simulink model "bh_3LINK_NEWTON_model_write_hello"  (R2022b)
settings: Solver=ode15s  StartTime=0.0  StopTime=30  FixedStep=0.001  RelTol=1e-6  EnableMultiTasking=on
libraries: sm_lib x1
settings Model: Creator=bhorton  LastModifiedBy=bhorton
settings SolverCC: ZeroCrossAlgorithm=Adaptive  AlgebraicLoopSolver=TrustRegion
settings DataIOCC: ReturnWorkspaceOutputs=off
settings OptimizationCC: BlockReduction=off  LifeSpan=inf
settings DebuggingCC: UnconnectedInputMsg=warning  UnconnectedOutputMsg=warning  UnconnectedLineMsg=warning  SFUnexpectedBacktrackingDiag=warning  SFNoUnconditionalDefaultTransitionDiag=warning  SFExecutionAtInitializationDiag=none  SFMachineParentedDataDiag=warning  ArithmeticOperatorsInVariantConditions=warning
settings ModelReferenceCC: EnableRefExpFcnMdlSchedulingChecks=on
settings SFSimCC: SimUseLocalCustomCode=off  CustomCodeUndefinedFunction=UseInterfaceOnly
settings RTWCC: RTWUseLocalCustomCode=off  DLArmComputeVersion=19.05
settings CodeAppCC: StateflowObjectComments=on
settings GRTTargetCC: TargetLangStandard=C89/C90 (ANSI)
settings ConfigComp: CovMetricSettings=dw  CovSaveCumulativeToWorkspaceVar=on  CovSaveSingleToWorkspaceVar=on  CovExternalEMLEnable=off
settings SimscapeCC: SimscapeNormalizeSystem=off  SimscapeLogType=all  SimscapeLogDataHistory=10000
settings ExplorerConfigSet: InternalSimMechanicsExplorerSettings="<ExplorerConfiguration><canonicalview>default</canonicalview><AnimationSetting><BasePlaybackSpeed>1.0</BasePlaybackSpeed><PlaybackSpeedFactor>1.0</PlaybackSpeedFactor></AnimationSetting><TilePanel><TileInfo><Tiles Columns=\"1\" Count=\"1\" Rows=\"1\"><Column Weight=\"1\"/><Row Weight=\"1\"/><Tile Height=\"1\" Width=\"1\" X=\"0\" Y=\"0\"/></Tiles></TileInfo><SceneInfo><SceneViewer><BGColor><R>0.60000002384185791</R><G>0.60000002384185791</G><B>0.60000002384185791</B></BGColor><Camera><DoPerspective>off</DoPerspective><Position><X>0.59337591503002618</X><Y>0.770028921233025243</Y><Z>1.16558506746291179</Z></Position><Center><X>0.554818716269093848</X><Y>0.595850240273192444</Y><Z>-0.00768042407463245119</Z></Center><Up><X>0.010293767731727228</X><Y>0.989057625734068191</Y><Z>-0.147170144129760788</Z></Up><ViewLimDist>1</ViewLimDist><YLim>0.684058578463238476</YLim><XLim>1.00632617542814184</XLim></Camera></SceneViewer></SceneInfo></TilePanel><MechEditorPanel><Cameras/><GfxPanelCameraMap/><VideoCreator><PlaybackSpeedRatio>1.0</PlaybackSpeedRatio><FrameRate>24</FrameRate><VideoFormat>MPEG-4</VideoFormat><FrameSize>[400 400]</FrameSize></VideoCreator></MechEditorPanel></ExplorerConfiguration>"

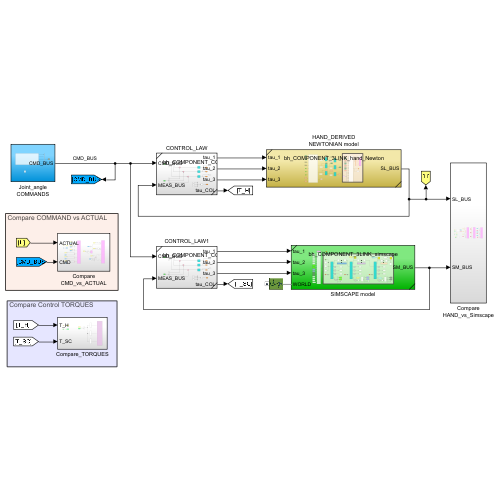
[thumbnail: Simulink's stored preview of the top-level diagram]
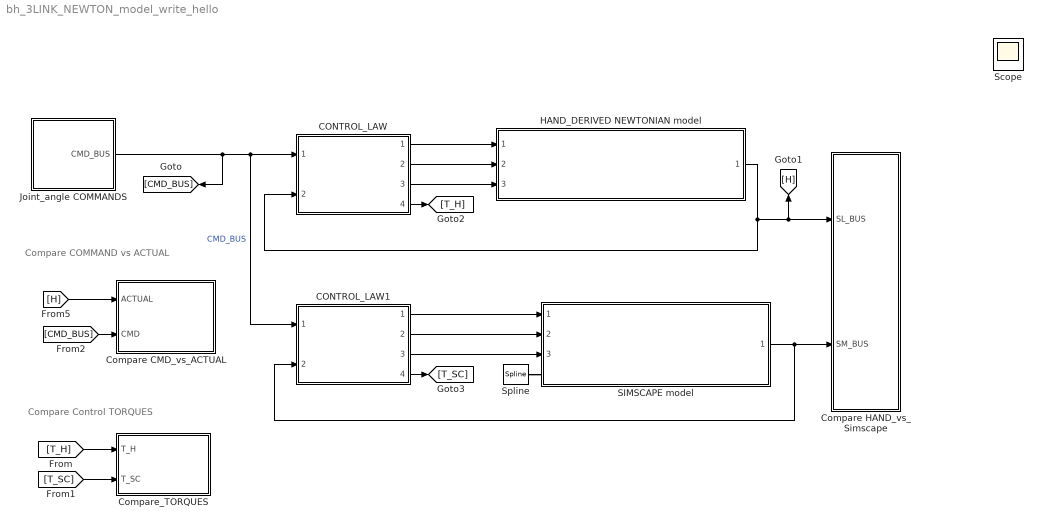
== system bh_3LINK_NEWTON_model_write_hello ==
  note: Compare Control TORQUES
  note: Compare COMMAND vs ACTUAL
  CONTROL_LAW : Subsystem  ReferencedSubsystem=bh_COMPONENT_CONTROL_LAW
  CONTROL_LAW1 : Subsystem  ReferencedSubsystem=bh_COMPONENT_CONTROL_LAW
  Compare CMD_vs_ACTUAL : Subsystem
  Compare HAND_vs_Simscape : Subsystem
  Compare_TORQUES : Subsystem
  HAND_DERIVED NEWTONIAN model : Subsystem  ReferencedSubsystem=bh_COMPONENT_3LINK_hand_Newton
  Joint_angle COMMANDS : Subsystem
  SIMSCAPE model : Subsystem  ReferencedSubsystem=bh_COMPONENT_3LINK_simscape
  Spline : sm_lib/Curves and Surfaces/Spline  GraphicAmbientColor=[0.15 0.15 0.15 1.0]  GraphicDiffuseColor=[0.0 1.0 0.0]  DataPoints=the_EE.XYZ_spline  DataPointsUnits=m  GraphicEmissiveColor=[0.0 0.0 0.0 1.0]  EndConditionType=Natural  MarkerShape=Sphere  MarkerSize=10  GraphicType=FromGeometry  GraphicOpacity=1.0  GraphicShininess=75  GraphicSpecularColor=[0.5 0.5 0.5 1.0]  GraphicVisPropType=SimpleVisualProperties
  Scope : Scope
  wires:
  SIMSCAPE model/1 -> CONTROL_LAW1/2, Compare HAND_vs_Simscape/2(SM_BUS)
  HAND_DERIVED NEWTONIAN model/1 -> Compare HAND_vs_Simscape/1(SL_BUS), [H], CONTROL_LAW/2
  Joint_angle COMMANDS/1(CMD_BUS) -> [CMD_BUS], CONTROL_LAW1/1, CONTROL_LAW/1  "CMD_BUS"
  CONTROL_LAW/1 -> HAND_DERIVED NEWTONIAN model/1
  CONTROL_LAW/2 -> HAND_DERIVED NEWTONIAN model/2
  CONTROL_LAW/3 -> HAND_DERIVED NEWTONIAN model/3
  CONTROL_LAW1/1 -> SIMSCAPE model/1
  CONTROL_LAW1/2 -> SIMSCAPE model/2
  CONTROL_LAW1/3 -> SIMSCAPE model/3
  [CMD_BUS] -> Compare CMD_vs_ACTUAL/2(CMD)
  [H] -> Compare CMD_vs_ACTUAL/1(ACTUAL)
  CONTROL_LAW/4 -> [T_H]
  CONTROL_LAW1/4 -> [T_SC]
  [T_SC] -> Compare_TORQUES/2(T_SC)
  [T_H] -> Compare_TORQUES/1(T_H)
  connections:
  Spline/LConn1 -- SIMSCAPE model/LConn1

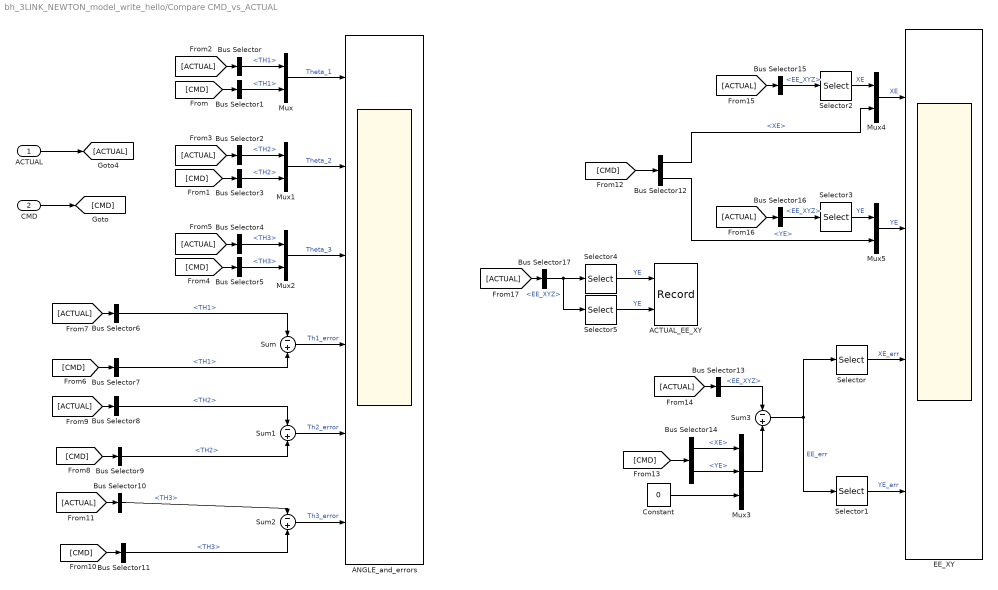
== system bh_3LINK_NEWTON_model_write_hello/Compare CMD_vs_ACTUAL ==
  ACTUAL : Inport
  CMD : Inport  Port=2
  ACTUAL_EE_XY : Record  FileSettingsInternal="{\"entries\":[{\"content\":{\"excelSettings\":{\"content\":{},\"type\":\"Streamout.ExcelSettings\"}},\"type\":\"Streamout.FileSettingStorage\",\"uuid\":\"47bc9f06-3dd7-4c30-9e65-8a4f675568b5\"}],\"packageUris\":[\"http://schema.mathworks.com/mf0/streamout_blocks/R2020a\"],\"version\":\"1.0\"}"  Layout=[1 1]  SignalsInternal="{\"entries\":[{\"content\":{\"signals\":[{\"content\":{\"blockPath\":[\"bh_3LINK_NEWTON_model_write_hello/Compare CMD_vs_ACTUAL/ACTUAL_EE_XY\"],\"channel\":[],\"dimensions\":[1],\"domain\":\"bh_3LINK_NEWTON_model_write_hello/Compare CMD_vs_ACTUAL/ACTUAL_EE_XY\",\"lineColor\":\"#ff6929\",\"plots\":[],\"port\":1,\"sid\":[],\"signalID\":3905,\"signalName\":\"YE\"},\"type\":\"RecordBlkView.Signal\",\"uuid\":\"7d422940-e755-4ad5-abac-504df8c7a942\"},{\"content\":{\"blockPath\":[\"bh_3LINK_NEWTON_model_write_hello/Compare CMD_vs_ACTUAL/ACTUAL_EE_XY\"],\"channel\":[],\"dimensions\":[1],\"domain\":\"bh_3LINK_NEWTON_model_write_hello/Compare CMD_vs_ACTUAL/ACTUAL_EE_XY\",\"lineColor\":\"#b746ff\",\"plots\":[],\"port\":2,\"sid\":[],\"signalID\":3908,\"signalName\":\"YE\"},\"type\":\"RecordBlkView.Signal\",\"uuid\":\"e4267c01-9c27-4ae9-8327-b877059776d0\"}]},\"type\":\"RecordBlkView.InputSignals\",\"uuid\":\"38542130-8fed-4a5c-a1bf-593c8935b6a0\"}],\"packageUris\":[\"http://schema.mathworks.com/mf0/streamout_blocks/R2020a\"],\"version\":\"1.0\"}"  VisualizationBindings="{\"xyplotplugin\":{\"info\":[{\"series\":[],\"subplotID\":1}]}}"  CompatibilityTag=XY  st=-1
  ANGLE_and_errors : Scope  NumInputPorts=6
  Bus Selector{,1,6..7} (4 alike) : BusSelector  OutputSignals=TH1
  Bus Selector{4..5,10..11} (4 alike) : BusSelector  OutputSignals=TH3
  Bus Selector12 : BusSelector  OutputSignals=XE,YE
  Bus Selector{13,15..17} (4 alike) : BusSelector  OutputSignals=EE_XYZ
  Bus Selector14 : BusSelector  OutputSignals=XE,YE
  Bus Selector{2..3,8..9} (4 alike) : BusSelector  OutputSignals=TH2
  Constant : Constant  Value=0
  EE_XY : Scope  NumInputPorts=4
  Mux{,1..2,4..5} (5 alike) : Mux  Inputs=2
  Mux3 : Mux  Inputs=3
  Selector : Selector  InputPortWidth=3  IndexOptions=Index vector (dialog)  Indices=1  OutputSizes=1
  Selector1 : Selector  InputPortWidth=3  IndexOptions=Index vector (dialog)  Indices=2  OutputSizes=1
  Selector2 : Selector  InputPortWidth=3  IndexOptions=Index vector (dialog)  Indices=1  OutputSizes=1
  Selector3 : Selector  InputPortWidth=3  IndexOptions=Index vector (dialog)  Indices=2  OutputSizes=1
  Selector4 : Selector  InputPortWidth=3  IndexOptions=Index vector (dialog)  Indices=1  OutputSizes=1
  Selector5 : Selector  InputPortWidth=3  IndexOptions=Index vector (dialog)  Indices=2  OutputSizes=1
  Sum{,1..3} (4 alike) : Sum  Inputs=-|+
  wires:
  ACTUAL/1 -> [ACTUAL]
  CMD/1 -> [CMD]
  [ACTUAL] -> Bus Selector/1
  Mux/1 -> ANGLE_and_errors/1  "Theta_1"
  Bus Selector/1 -> Mux/1  "<TH1>"
  [CMD] -> Bus Selector1/1
  Bus Selector1/1 -> Mux/2  "<TH1>"
  Bus Selector3/1 -> Mux1/2  "<TH2>"
  [CMD] -> Bus Selector3/1
  Mux1/1 -> ANGLE_and_errors/2  "Theta_2"
  [ACTUAL] -> Bus Selector2/1
  Bus Selector2/1 -> Mux1/1  "<TH2>"
  Mux2/1 -> ANGLE_and_errors/3  "Theta_3"
  [ACTUAL] -> Bus Selector4/1
  [CMD] -> Bus Selector5/1
  Bus Selector5/1 -> Mux2/2  "<TH3>"
  Bus Selector4/1 -> Mux2/1  "<TH3>"
  Sum/1 -> ANGLE_and_errors/4  "Th1_error"
  Sum1/1 -> ANGLE_and_errors/5  "Th2_error"
  Sum2/1 -> ANGLE_and_errors/6  "Th3_error"
  Bus Selector7/1 -> Sum/2  "<TH1>"
  [CMD] -> Bus Selector7/1
  [ACTUAL] -> Bus Selector6/1
  Bus Selector6/1 -> Sum/1  "<TH1>"
  [ACTUAL] -> Bus Selector8/1
  [CMD] -> Bus Selector9/1
  Bus Selector9/1 -> Sum1/2  "<TH2>"
  Bus Selector8/1 -> Sum1/1  "<TH2>"
  Bus Selector11/1 -> Sum2/2  "<TH3>"
  [ACTUAL] -> Bus Selector10/1
  Bus Selector10/1 -> Sum2/1  "<TH3>"
  [CMD] -> Bus Selector11/1
  [CMD] -> Bus Selector12/1
  [ACTUAL] -> Bus Selector13/1
  [CMD] -> Bus Selector14/1
  Sum3/1 -> Selector1/1, Selector/1  "EE_err"
  Selector1/1 -> EE_XY/4  "YE_err"
  Selector/1 -> EE_XY/3  "XE_err"
  Constant/1 -> Mux3/3
  Bus Selector14/1 -> Mux3/1  "<XE>"
  Bus Selector14/2 -> Mux3/2  "<YE>"
  Mux3/1 -> Sum3/2
  Bus Selector13/1 -> Sum3/1  "<EE_XYZ>"
  [ACTUAL] -> Bus Selector15/1
  Bus Selector15/1 -> Selector2/1  "<EE_XYZ>"
  Mux4/1 -> EE_XY/1  "XE"
  Selector2/1 -> Mux4/1  "XE"
  Bus Selector12/1 -> Mux4/2  "<XE>"
  [ACTUAL] -> Bus Selector16/1
  Bus Selector16/1 -> Selector3/1  "<EE_XYZ>"
  Selector3/1 -> Mux5/1  "YE"
  Mux5/1 -> EE_XY/2  "YE"
  Bus Selector12/2 -> Mux5/2  "<YE>"
  [ACTUAL] -> Bus Selector17/1
  Bus Selector17/1 -> Selector5/1, Selector4/1  "<EE_XYZ>"
  Selector5/1 -> ACTUAL_EE_XY/2  "YE"
  Selector4/1 -> ACTUAL_EE_XY/1  "YE"

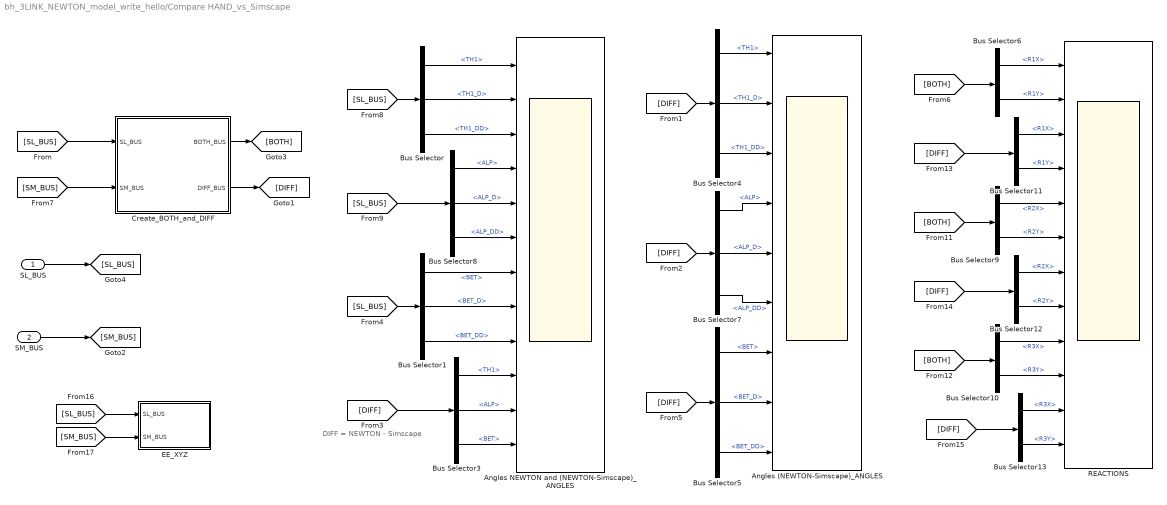
== system bh_3LINK_NEWTON_model_write_hello/Compare HAND_vs_Simscape ==
  note: DIFF = NEWTON - Simscape
  SL_BUS : Inport
  SM_BUS : Inport  Port=2
  Angles (NEWTON-Simscape)_ANGLES : Scope  NumInputPorts=9
  Angles NEWTON and (NEWTON-Simscape)_ANGLES : Scope  NumInputPorts=12
  Bus Selector : BusSelector  OutputSignals=TH1,TH1_D,TH1_DD
  Bus Selector1 : BusSelector  OutputSignals=BET,BET_D,BET_DD
  Bus Selector10 : BusSelector  OutputSignals=R3X,R3Y
  Bus Selector11 : BusSelector  OutputSignals=R1X,R1Y
  Bus Selector12 : BusSelector  OutputSignals=R2X,R2Y
  Bus Selector13 : BusSelector  OutputSignals=R3X,R3Y
  Bus Selector3 : BusSelector  OutputSignals=TH1,ALP,BET
  Bus Selector4 : BusSelector  OutputSignals=TH1,TH1_D,TH1_DD
  Bus Selector5 : BusSelector  OutputSignals=BET,BET_D,BET_DD
  Bus Selector6 : BusSelector  OutputSignals=R1X,R1Y
  Bus Selector7 : BusSelector  OutputSignals=ALP,ALP_D,ALP_DD
  Bus Selector8 : BusSelector  OutputSignals=ALP,ALP_D,ALP_DD
  Bus Selector9 : BusSelector  OutputSignals=R2X,R2Y
  Create_BOTH_and_DIFF : Subsystem
  EE_XYZ : Subsystem
  REACTIONS : Scope  NumInputPorts=12
  wires:
  [SM_BUS] -> Create_BOTH_and_DIFF/2(SM_BUS)
  Bus Selector/3 -> Angles NEWTON and (NEWTON-Simscape)_ANGLES/3  "<TH1_DD>"
  Bus Selector/2 -> Angles NEWTON and (NEWTON-Simscape)_ANGLES/2  "<TH1_D>"
  Bus Selector/1 -> Angles NEWTON and (NEWTON-Simscape)_ANGLES/1  "<TH1>"
  [SL_BUS] -> Create_BOTH_and_DIFF/1(SL_BUS)
  Bus Selector8/1 -> Angles NEWTON and (NEWTON-Simscape)_ANGLES/4  "<ALP>"
  Bus Selector8/2 -> Angles NEWTON and (NEWTON-Simscape)_ANGLES/5  "<ALP_D>"
  Bus Selector8/3 -> Angles NEWTON and (NEWTON-Simscape)_ANGLES/6  "<ALP_DD>"
  Bus Selector1/1 -> Angles NEWTON and (NEWTON-Simscape)_ANGLES/7  "<BET>"
  Bus Selector1/2 -> Angles NEWTON and (NEWTON-Simscape)_ANGLES/8  "<BET_D>"
  Bus Selector1/3 -> Angles NEWTON and (NEWTON-Simscape)_ANGLES/9  "<BET_DD>"
  Bus Selector3/1 -> Angles NEWTON and (NEWTON-Simscape)_ANGLES/10  "<TH1>"
  Bus Selector3/2 -> Angles NEWTON and (NEWTON-Simscape)_ANGLES/11  "<ALP>"
  Bus Selector3/3 -> Angles NEWTON and (NEWTON-Simscape)_ANGLES/12  "<BET>"
  Create_BOTH_and_DIFF/1(BOTH_BUS) -> [BOTH]
  Create_BOTH_and_DIFF/2(DIFF_BUS) -> [DIFF]
  [SL_BUS] -> Bus Selector/1
  [DIFF] -> Bus Selector3/1
  SL_BUS/1 -> [SL_BUS]
  SM_BUS/1 -> [SM_BUS]
  [SL_BUS] -> Bus Selector8/1
  [SL_BUS] -> Bus Selector1/1
  [DIFF] -> Bus Selector5/1
  [DIFF] -> Bus Selector7/1
  Bus Selector7/3 -> Angles (NEWTON-Simscape)_ANGLES/6  "<ALP_DD>"
  Bus Selector5/3 -> Angles (NEWTON-Simscape)_ANGLES/9  "<BET_DD>"
  [DIFF] -> Bus Selector4/1
  Bus Selector4/1 -> Angles (NEWTON-Simscape)_ANGLES/1  "<TH1>"
  Bus Selector4/3 -> Angles (NEWTON-Simscape)_ANGLES/3  "<TH1_DD>"
  Bus Selector5/1 -> Angles (NEWTON-Simscape)_ANGLES/7  "<BET>"
  Bus Selector7/2 -> Angles (NEWTON-Simscape)_ANGLES/5  "<ALP_D>"
  Bus Selector5/2 -> Angles (NEWTON-Simscape)_ANGLES/8  "<BET_D>"
  Bus Selector7/1 -> Angles (NEWTON-Simscape)_ANGLES/4  "<ALP>"
  Bus Selector4/2 -> Angles (NEWTON-Simscape)_ANGLES/2  "<TH1_D>"
  [BOTH] -> Bus Selector6/1
  Bus Selector6/1 -> REACTIONS/1  "<R1X>"
  Bus Selector6/2 -> REACTIONS/2  "<R1Y>"
  Bus Selector9/1 -> REACTIONS/5  "<R2X>"
  Bus Selector9/2 -> REACTIONS/6  "<R2Y>"
  [BOTH] -> Bus Selector9/1
  [BOTH] -> Bus Selector10/1
  Bus Selector10/1 -> REACTIONS/9  "<R3X>"
  Bus Selector10/2 -> REACTIONS/10  "<R3Y>"
  [DIFF] -> Bus Selector11/1
  Bus Selector11/1 -> REACTIONS/3  "<R1X>"
  Bus Selector11/2 -> REACTIONS/4  "<R1Y>"
  [DIFF] -> Bus Selector12/1
  Bus Selector12/1 -> REACTIONS/7  "<R2X>"
  Bus Selector12/2 -> REACTIONS/8  "<R2Y>"
  [DIFF] -> Bus Selector13/1
  Bus Selector13/1 -> REACTIONS/11  "<R3X>"
  Bus Selector13/2 -> REACTIONS/12  "<R3Y>"
  [SL_BUS] -> EE_XYZ/1(SL_BUS)
  [SM_BUS] -> EE_XYZ/2(SM_BUS)

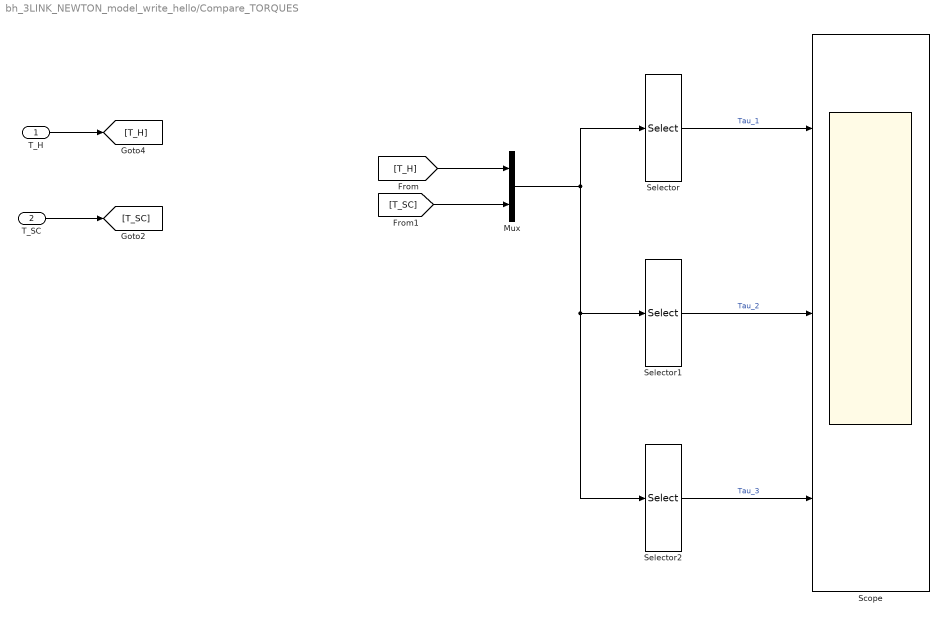
== system bh_3LINK_NEWTON_model_write_hello/Compare_TORQUES ==
  T_H : Inport
  T_SC : Inport  Port=2
  Mux : Mux  Inputs=2
  Scope : Scope  NumInputPorts=3
  Selector : Selector  InputPortWidth=6  IndexOptions=Index vector (dialog)  Indices=[1,4]  OutputSizes=1
  Selector1 : Selector  InputPortWidth=6  IndexOptions=Index vector (dialog)  Indices=[2,5]  OutputSizes=1
  Selector2 : Selector  InputPortWidth=6  IndexOptions=Index vector (dialog)  Indices=[3,6]  OutputSizes=1
  wires:
  T_H/1 -> [T_H]
  T_SC/1 -> [T_SC]
  [T_H] -> Mux/1
  [T_SC] -> Mux/2
  Mux/1 -> Selector2/1, Selector1/1, Selector/1
  Selector/1 -> Scope/1  "Tau_1"
  Selector1/1 -> Scope/2  "Tau_2"
  Selector2/1 -> Scope/3  "Tau_3"

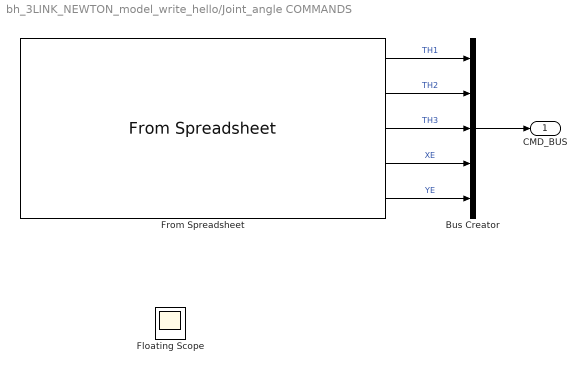
== system bh_3LINK_NEWTON_model_write_hello/Joint_angle COMMANDS ==
  Bus Creator : BusCreator  Inputs=5
  Floating Scope : Scope
      settings: Floating=on
  From Spreadsheet : FromSpreadsheet  FileName=TRAJECTORY_DATA_3LINK.xlsx  SheetName=T_TH_XY  ExtrapolationAfterLastDataPoint=Hold last value
  CMD_BUS : Outport
  wires:
  Bus Creator/1 -> CMD_BUS/1
  From Spreadsheet/1 -> Bus Creator/1  "TH1"
  From Spreadsheet/2 -> Bus Creator/2  "TH2"
  From Spreadsheet/3 -> Bus Creator/3  "TH3"
  From Spreadsheet/4 -> Bus Creator/4  "XE"
  From Spreadsheet/5 -> Bus Creator/5  "YE"

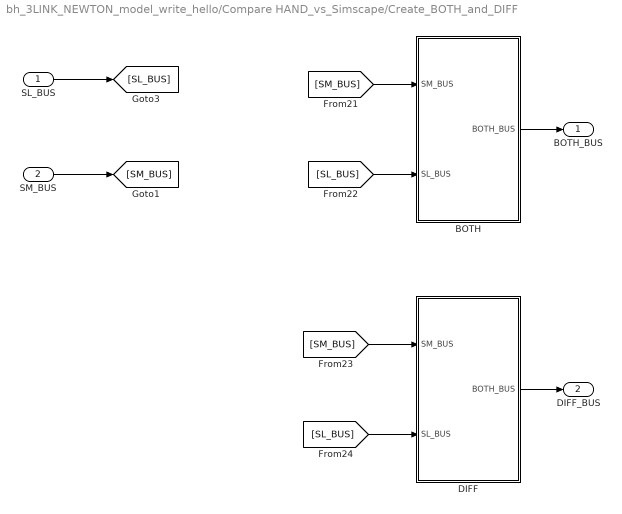
== system bh_3LINK_NEWTON_model_write_hello/Compare HAND_vs_Simscape/Create_BOTH_and_DIFF ==
  SL_BUS : Inport
  SM_BUS : Inport  Port=2
  BOTH : Subsystem
  DIFF : Subsystem
  BOTH_BUS : Outport
  DIFF_BUS : Outport  Port=2
  wires:
  SL_BUS/1 -> [SL_BUS]
  SM_BUS/1 -> [SM_BUS]
  [SM_BUS] -> BOTH/1(SM_BUS)
  [SL_BUS] -> BOTH/2(SL_BUS)
  [SM_BUS] -> DIFF/1(SM_BUS)
  [SL_BUS] -> DIFF/2(SL_BUS)
  DIFF/1(BOTH_BUS) -> DIFF_BUS/1
  BOTH/1(BOTH_BUS) -> BOTH_BUS/1

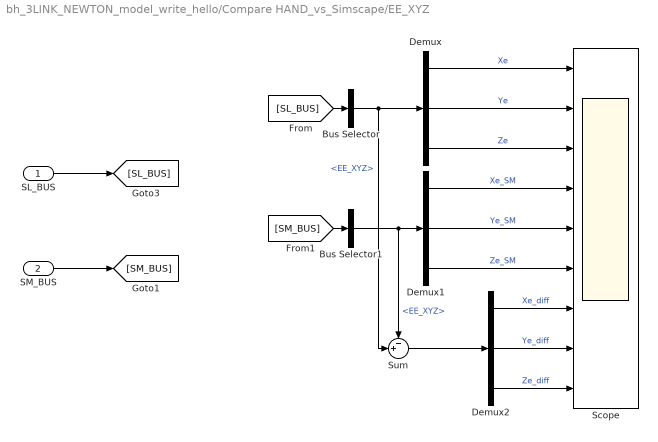
== system bh_3LINK_NEWTON_model_write_hello/Compare HAND_vs_Simscape/EE_XYZ ==
  SL_BUS : Inport
  SM_BUS : Inport  Port=2
  Bus Selector : BusSelector  OutputSignals=EE_XYZ
  Bus Selector1 : BusSelector  OutputSignals=EE_XYZ
  Demux : Demux  Outputs=3
  Demux1 : Demux  Outputs=3
  Demux2 : Demux  Outputs=3
  Scope : Scope  NumInputPorts=9
  Sum : Sum  Inputs=-+|
  wires:
  SM_BUS/1 -> [SM_BUS]
  SL_BUS/1 -> [SL_BUS]
  [SL_BUS] -> Bus Selector/1
  Demux/3 -> Scope/3  "Ze"
  Demux/2 -> Scope/2  "Ye"
  Demux/1 -> Scope/1  "Xe"
  Bus Selector/1 -> Sum/2, Demux/1  "<EE_XYZ>"
  [SM_BUS] -> Bus Selector1/1
  Bus Selector1/1 -> Sum/1, Demux1/1  "<EE_XYZ>"
  Demux1/2 -> Scope/5  "Ye_SM"
  Demux1/1 -> Scope/4  "Xe_SM"
  Demux1/3 -> Scope/6  "Ze_SM"
  Sum/1 -> Demux2/1
  Demux2/1 -> Scope/7  "Xe_diff"
  Demux2/2 -> Scope/8  "Ye_diff"
  Demux2/3 -> Scope/9  "Ze_diff"

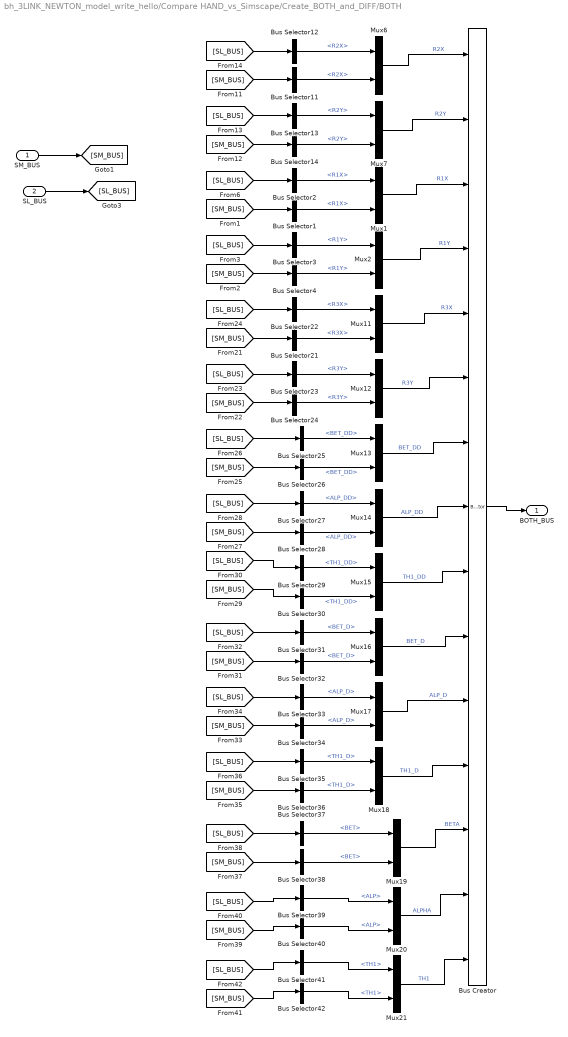
== system bh_3LINK_NEWTON_model_write_hello/Compare HAND_vs_Simscape/Create_BOTH_and_DIFF/BOTH ==
  SM_BUS : Inport
  SL_BUS : Inport  Port=2
  Bus Creator : BusCreator  Inputs=15
  Bus Selector1 : BusSelector  OutputSignals=R1X
  Bus Selector11 : BusSelector  OutputSignals=R2X
  Bus Selector12 : BusSelector  OutputSignals=R2X
  Bus Selector13 : BusSelector  OutputSignals=R2Y
  Bus Selector14 : BusSelector  OutputSignals=R2Y
  Bus Selector2 : BusSelector  OutputSignals=R1X
  Bus Selector21 : BusSelector  OutputSignals=R3X
  Bus Selector22 : BusSelector  OutputSignals=R3X
  Bus Selector23 : BusSelector  OutputSignals=R3Y
  Bus Selector24 : BusSelector  OutputSignals=R3Y
  Bus Selector25 : BusSelector  OutputSignals=BET_DD
  Bus Selector26 : BusSelector  OutputSignals=BET_DD
  Bus Selector27 : BusSelector  OutputSignals=ALP_DD
  Bus Selector28 : BusSelector  OutputSignals=ALP_DD
  Bus Selector29 : BusSelector  OutputSignals=TH1_DD
  Bus Selector3 : BusSelector  OutputSignals=R1Y
  Bus Selector30 : BusSelector  OutputSignals=TH1_DD
  Bus Selector31 : BusSelector  OutputSignals=BET_D
  Bus Selector32 : BusSelector  OutputSignals=BET_D
  Bus Selector33 : BusSelector  OutputSignals=ALP_D
  Bus Selector34 : BusSelector  OutputSignals=ALP_D
  Bus Selector35 : BusSelector  OutputSignals=TH1_D
  Bus Selector36 : BusSelector  OutputSignals=TH1_D
  Bus Selector37 : BusSelector  OutputSignals=BET
  Bus Selector38 : BusSelector  OutputSignals=BET
  Bus Selector39 : BusSelector  OutputSignals=ALP
  Bus Selector4 : BusSelector  OutputSignals=R1Y
  Bus Selector40 : BusSelector  OutputSignals=ALP
  Bus Selector41 : BusSelector  OutputSignals=TH1
  Bus Selector42 : BusSelector  OutputSignals=TH1
  Mux{1..2,6..7,11..21} (15 alike) : Mux  Inputs=2
  BOTH_BUS : Outport
  wires:
  SL_BUS/1 -> [SL_BUS]
  SM_BUS/1 -> [SM_BUS]
  [SL_BUS] -> Bus Selector2/1
  [SM_BUS] -> Bus Selector1/1
  [SL_BUS] -> Bus Selector3/1
  [SM_BUS] -> Bus Selector4/1
  Bus Selector1/1 -> Mux1/2  "<R1X>"
  Bus Selector2/1 -> Mux1/1  "<R1X>"
  Bus Selector3/1 -> Mux2/1  "<R1Y>"
  Bus Selector4/1 -> Mux2/2  "<R1Y>"
  Mux1/1 -> Bus Creator/3  "R1X"
  Mux2/1 -> Bus Creator/4  "R1Y"
  Bus Creator/1 -> BOTH_BUS/1
  [SL_BUS] -> Bus Selector12/1
  [SM_BUS] -> Bus Selector11/1
  [SL_BUS] -> Bus Selector13/1
  Bus Selector11/1 -> Mux6/2  "<R2X>"
  Bus Selector12/1 -> Mux6/1  "<R2X>"
  Bus Selector13/1 -> Mux7/1  "<R2Y>"
  Mux6/1 -> Bus Creator/1  "R2X"
  Mux7/1 -> Bus Creator/2  "R2Y"
  [SM_BUS] -> Bus Selector14/1
  Bus Selector14/1 -> Mux7/2  "<R2Y>"
  Mux11/1 -> Bus Creator/5  "R3X"
  Bus Selector24/1 -> Mux12/2  "<R3Y>"
  Mux12/1 -> Bus Creator/6  "R3Y"
  Bus Selector23/1 -> Mux12/1  "<R3Y>"
  [SL_BUS] -> Bus Selector23/1
  [SM_BUS] -> Bus Selector24/1
  [SM_BUS] -> Bus Selector21/1
  Bus Selector22/1 -> Mux11/1  "<R3X>"
  Bus Selector21/1 -> Mux11/2  "<R3X>"
  [SL_BUS] -> Bus Selector22/1
  Mux13/1 -> Bus Creator/7  "BET_DD"
  Mux14/1 -> Bus Creator/8  "ALP_DD"
  Mux15/1 -> Bus Creator/9  "TH1_DD"
  Mux16/1 -> Bus Creator/10  "BET_D"
  Mux18/1 -> Bus Creator/12  "TH1_D"
  Mux17/1 -> Bus Creator/11  "ALP_D"
  Mux20/1 -> Bus Creator/14  "ALPHA"
  Mux19/1 -> Bus Creator/13  "BETA"
  Mux21/1 -> Bus Creator/15  "TH1"
  [SL_BUS] -> Bus Selector25/1
  [SM_BUS] -> Bus Selector26/1
  [SL_BUS] -> Bus Selector27/1
  [SM_BUS] -> Bus Selector28/1
  [SL_BUS] -> Bus Selector29/1
  [SM_BUS] -> Bus Selector30/1
  [SL_BUS] -> Bus Selector31/1
  [SM_BUS] -> Bus Selector32/1
  [SL_BUS] -> Bus Selector33/1
  [SM_BUS] -> Bus Selector34/1
  [SL_BUS] -> Bus Selector35/1
  [SM_BUS] -> Bus Selector36/1
  [SL_BUS] -> Bus Selector37/1
  [SM_BUS] -> Bus Selector38/1
  [SL_BUS] -> Bus Selector39/1
  [SM_BUS] -> Bus Selector40/1
  [SL_BUS] -> Bus Selector41/1
  [SM_BUS] -> Bus Selector42/1
  Bus Selector25/1 -> Mux13/1  "<BET_DD>"
  Bus Selector26/1 -> Mux13/2  "<BET_DD>"
  Bus Selector27/1 -> Mux14/1  "<ALP_DD>"
  Bus Selector28/1 -> Mux14/2  "<ALP_DD>"
  Bus Selector29/1 -> Mux15/1  "<TH1_DD>"
  Bus Selector30/1 -> Mux15/2  "<TH1_DD>"
  Bus Selector32/1 -> Mux16/2  "<BET_D>"
  Bus Selector31/1 -> Mux16/1  "<BET_D>"
  Bus Selector33/1 -> Mux17/1  "<ALP_D>"
  Bus Selector34/1 -> Mux17/2  "<ALP_D>"
  Bus Selector35/1 -> Mux18/1  "<TH1_D>"
  Bus Selector36/1 -> Mux18/2  "<TH1_D>"
  Bus Selector37/1 -> Mux19/1  "<BET>"
  Bus Selector38/1 -> Mux19/2  "<BET>"
  Bus Selector39/1 -> Mux20/1  "<ALP>"
  Bus Selector40/1 -> Mux20/2  "<ALP>"
  Bus Selector42/1 -> Mux21/2  "<TH1>"
  Bus Selector41/1 -> Mux21/1  "<TH1>"

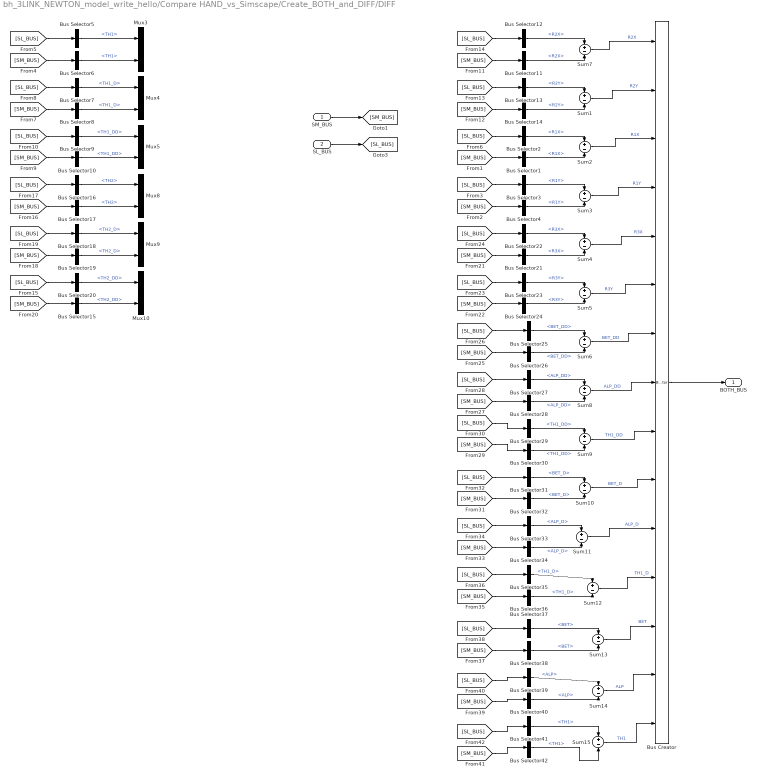
== system bh_3LINK_NEWTON_model_write_hello/Compare HAND_vs_Simscape/Create_BOTH_and_DIFF/DIFF ==
  SM_BUS : Inport
  SL_BUS : Inport  Port=2
  Bus Creator : BusCreator  Inputs=15
  Bus Selector1 : BusSelector  OutputSignals=R1X
  Bus Selector{9..10,29..30} (4 alike) : BusSelector  OutputSignals=TH1_DD
  Bus Selector11 : BusSelector  OutputSignals=R2X
  Bus Selector12 : BusSelector  OutputSignals=R2X
  Bus Selector13 : BusSelector  OutputSignals=R2Y
  Bus Selector14 : BusSelector  OutputSignals=R2Y
  Bus Selector15 : BusSelector  OutputSignals=TH2_DD
  Bus Selector16 : BusSelector  OutputSignals=TH2
  Bus Selector17 : BusSelector  OutputSignals=TH2
  Bus Selector18 : BusSelector  OutputSignals=TH2_D
  Bus Selector19 : BusSelector  OutputSignals=TH2_D
  Bus Selector2 : BusSelector  OutputSignals=R1X
  Bus Selector20 : BusSelector  OutputSignals=TH2_DD
  Bus Selector21 : BusSelector  OutputSignals=R3X
  Bus Selector22 : BusSelector  OutputSignals=R3X
  Bus Selector23 : BusSelector  OutputSignals=R3Y
  Bus Selector24 : BusSelector  OutputSignals=R3Y
  Bus Selector25 : BusSelector  OutputSignals=BET_DD
  Bus Selector26 : BusSelector  OutputSignals=BET_DD
  Bus Selector27 : BusSelector  OutputSignals=ALP_DD
  Bus Selector28 : BusSelector  OutputSignals=ALP_DD
  Bus Selector3 : BusSelector  OutputSignals=R1Y
  Bus Selector31 : BusSelector  OutputSignals=BET_D
  Bus Selector32 : BusSelector  OutputSignals=BET_D
  Bus Selector33 : BusSelector  OutputSignals=ALP_D
  Bus Selector34 : BusSelector  OutputSignals=ALP_D
  Bus Selector{7..8,35..36} (4 alike) : BusSelector  OutputSignals=TH1_D
  Bus Selector37 : BusSelector  OutputSignals=BET
  Bus Selector38 : BusSelector  OutputSignals=BET
  Bus Selector39 : BusSelector  OutputSignals=ALP
  Bus Selector4 : BusSelector  OutputSignals=R1Y
  Bus Selector40 : BusSelector  OutputSignals=ALP
  Bus Selector{5..6,41..42} (4 alike) : BusSelector  OutputSignals=TH1
  Mux{3..5,8..10} (6 alike) : Mux  Inputs=2
  Sum{1..15} (15 alike) : Sum  Inputs=+|-
  BOTH_BUS : Outport
  wires:
  SL_BUS/1 -> [SL_BUS]
  SM_BUS/1 -> [SM_BUS]
  [SL_BUS] -> Bus Selector2/1
  [SM_BUS] -> Bus Selector1/1
  [SL_BUS] -> Bus Selector3/1
  [SM_BUS] -> Bus Selector4/1
  [SM_BUS] -> Bus Selector6/1
  [SL_BUS] -> Bus Selector5/1
  [SL_BUS] -> Bus Selector7/1
  [SM_BUS] -> Bus Selector8/1
  [SL_BUS] -> Bus Selector9/1
  [SM_BUS] -> Bus Selector10/1
  Bus Selector1/1 -> Sum2/2  "<R1X>"
  Bus Selector2/1 -> Sum2/1  "<R1X>"
  Bus Selector3/1 -> Sum3/1  "<R1Y>"
  Bus Selector4/1 -> Sum3/2  "<R1Y>"
  Bus Selector5/1 -> Mux3/1  "<TH1>"
  Bus Selector6/1 -> Mux3/2  "<TH1>"
  Bus Selector7/1 -> Mux4/1  "<TH1_D>"
  Bus Selector8/1 -> Mux4/2  "<TH1_D>"
  Bus Selector9/1 -> Mux5/1  "<TH1_DD>"
  Bus Selector10/1 -> Mux5/2  "<TH1_DD>"
  Sum2/1 -> Bus Creator/3  "R1X"
  Sum3/1 -> Bus Creator/4  "R1Y"
  Bus Creator/1 -> BOTH_BUS/1
  [SL_BUS] -> Bus Selector12/1
  [SM_BUS] -> Bus Selector11/1
  [SL_BUS] -> Bus Selector13/1
  Bus Selector11/1 -> Sum7/2  "<R2X>"
  Bus Selector12/1 -> Sum7/1  "<R2X>"
  Bus Selector13/1 -> Sum1/1  "<R2Y>"
  Sum7/1 -> Bus Creator/1  "R2X"
  Sum1/1 -> Bus Creator/2  "R2Y"
  [SM_BUS] -> Bus Selector14/1
  Bus Selector14/1 -> Sum1/2  "<R2Y>"
  [SM_BUS] -> Bus Selector17/1
  [SL_BUS] -> Bus Selector16/1
  [SL_BUS] -> Bus Selector18/1
  [SM_BUS] -> Bus Selector19/1
  [SL_BUS] -> Bus Selector20/1
  [SM_BUS] -> Bus Selector15/1
  Bus Selector16/1 -> Mux8/1  "<TH2>"
  Bus Selector17/1 -> Mux8/2  "<TH2>"
  Bus Selector18/1 -> Mux9/1  "<TH2_D>"
  Bus Selector19/1 -> Mux9/2  "<TH2_D>"
  Bus Selector20/1 -> Mux10/1  "<TH2_DD>"
  Bus Selector15/1 -> Mux10/2  "<TH2_DD>"
  Sum4/1 -> Bus Creator/5  "R3X"
  Bus Selector24/1 -> Sum5/2  "<R3Y>"
  Sum5/1 -> Bus Creator/6  "R3Y"
  Bus Selector23/1 -> Sum5/1  "<R3Y>"
  [SL_BUS] -> Bus Selector23/1
  [SM_BUS] -> Bus Selector24/1
  [SM_BUS] -> Bus Selector21/1
  Bus Selector22/1 -> Sum4/1  "<R3X>"
  Bus Selector21/1 -> Sum4/2  "<R3X>"
  [SL_BUS] -> Bus Selector22/1
  Sum6/1 -> Bus Creator/7  "BET_DD"
  Sum8/1 -> Bus Creator/8  "ALP_DD"
  Sum9/1 -> Bus Creator/9  "TH1_DD"
  Sum10/1 -> Bus Creator/10  "BET_D"
  Sum12/1 -> Bus Creator/12  "TH1_D"
  Sum11/1 -> Bus Creator/11  "ALP_D"
  Sum14/1 -> Bus Creator/14  "ALP"
  Sum13/1 -> Bus Creator/13  "BET"
  Sum15/1 -> Bus Creator/15  "TH1"
  [SL_BUS] -> Bus Selector25/1
  [SM_BUS] -> Bus Selector26/1
  [SL_BUS] -> Bus Selector27/1
  [SM_BUS] -> Bus Selector28/1
  [SL_BUS] -> Bus Selector29/1
  [SM_BUS] -> Bus Selector30/1
  [SL_BUS] -> Bus Selector31/1
  [SM_BUS] -> Bus Selector32/1
  [SL_BUS] -> Bus Selector33/1
  [SM_BUS] -> Bus Selector34/1
  [SL_BUS] -> Bus Selector35/1
  [SM_BUS] -> Bus Selector36/1
  [SL_BUS] -> Bus Selector37/1
  [SM_BUS] -> Bus Selector38/1
  [SL_BUS] -> Bus Selector39/1
  [SM_BUS] -> Bus Selector40/1
  [SL_BUS] -> Bus Selector41/1
  [SM_BUS] -> Bus Selector42/1
  Bus Selector25/1 -> Sum6/1  "<BET_DD>"
  Bus Selector26/1 -> Sum6/2  "<BET_DD>"
  Bus Selector27/1 -> Sum8/1  "<ALP_DD>"
  Bus Selector28/1 -> Sum8/2  "<ALP_DD>"
  Bus Selector29/1 -> Sum9/1  "<TH1_DD>"
  Bus Selector30/1 -> Sum9/2  "<TH1_DD>"
  Bus Selector32/1 -> Sum10/2  "<BET_D>"
  Bus Selector31/1 -> Sum10/1  "<BET_D>"
  Bus Selector33/1 -> Sum11/1  "<ALP_D>"
  Bus Selector34/1 -> Sum11/2  "<ALP_D>"
  Bus Selector35/1 -> Sum12/1  "<TH1_D>"
  Bus Selector36/1 -> Sum12/2  "<TH1_D>"
  Bus Selector37/1 -> Sum13/1  "<BET>"
  Bus Selector38/1 -> Sum13/2  "<BET>"
  Bus Selector39/1 -> Sum14/1  "<ALP>"
  Bus Selector40/1 -> Sum14/2  "<ALP>"
  Bus Selector42/1 -> Sum15/2  "<TH1>"
  Bus Selector41/1 -> Sum15/1  "<TH1>"
